simulink model "tau_10"  (R2019b)
settings: Solver=VariableStepAuto  StartTime=0.0  StopTime=10  RelTol=1e-3
model workspace (MAT data in the model file):
  k = 0.5
libraries: simulink x3
settings Model: Creator=Sergey  LastModifiedBy=Sergey

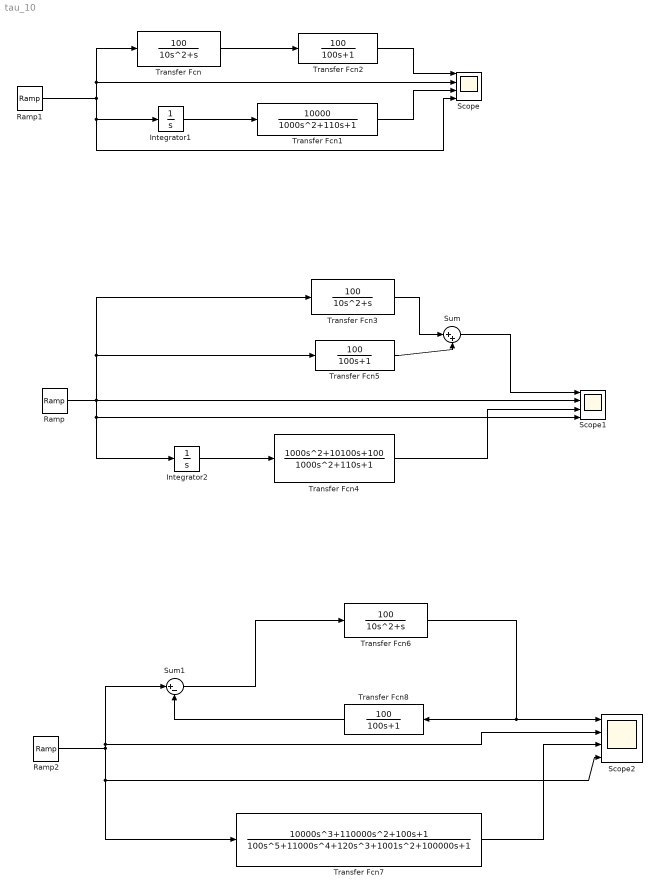
== system tau_10 ==
  Integrator1 : Integrator
  Integrator2 : Integrator
  Ramp : simulink/Sources/Ramp  slope=1  start=0  InitialOutput=0
  Ramp1 : simulink/Sources/Ramp  slope=1  start=0  InitialOutput=0
  Ramp2 : simulink/Sources/Ramp  slope=1  start=0  InitialOutput=0
  Scope : Scope  NumInputPorts=4
  Scope1 : Scope  NumInputPorts=4
  Scope2 : Scope  NumInputPorts=4
  Sum : Sum  Inputs=|++
  Sum1 : Sum  Inputs=|+-
  Transfer Fcn : TransferFcn  Numerator=[100]  Denominator=[10 1 0]
  Transfer Fcn1 : TransferFcn  Numerator=[10000]  Denominator=[1000 110 1]
  Transfer Fcn2 : TransferFcn  Numerator=[100]  Denominator=[100 1]
  Transfer Fcn3 : TransferFcn  Numerator=[100]  Denominator=[10 1 0]
  Transfer Fcn4 : TransferFcn  Numerator=[1000 10100 100]  Denominator=[1000 110 1]
  Transfer Fcn5 : TransferFcn  Numerator=[100]  Denominator=[100 1]
  Transfer Fcn6 : TransferFcn  Numerator=[100]  Denominator=[10 1 0]
  Transfer Fcn7 : TransferFcn  Numerator=[10000 110000 100 1]  Denominator=[100 11000 120 1001 100000 1]
  Transfer Fcn8 : TransferFcn  Numerator=[100]  Denominator=[100 1]
  wires:
  Ramp1/1 -> Transfer Fcn/1, Scope/2, Integrator1/1, Scope/4
  Transfer Fcn/1 -> Transfer Fcn2/1
  Integrator1/1 -> Transfer Fcn1/1
  Transfer Fcn2/1 -> Scope/1
  Transfer Fcn1/1 -> Scope/3
  Integrator2/1 -> Transfer Fcn4/1
  Ramp/1 -> Scope1/2, Integrator2/1, Scope1/4, Transfer Fcn5/1, Transfer Fcn3/1
  Transfer Fcn3/1 -> Sum/1
  Transfer Fcn5/1 -> Sum/2
  Sum/1 -> Scope1/1
  Transfer Fcn4/1 -> Scope1/3
  Transfer Fcn7/1 -> Scope2/3
  Ramp2/1 -> Sum1/1, Scope2/2, Transfer Fcn7/1, Scope2/4
  Transfer Fcn6/1 -> Transfer Fcn8/1, Scope2/1
  Transfer Fcn8/1 -> Sum1/2
  Sum1/1 -> Transfer Fcn6/1
